simulink subsystem "LeastCov_v3_5_adaptiveAlgorithm"  (R2022a)
settings: Solver=VariableStepAuto  StartTime=0.0  StopTime=10.0  RelTol=1e-3
libraries: simulink x2
settings Model: Creator=targi  LastModifiedBy=targi

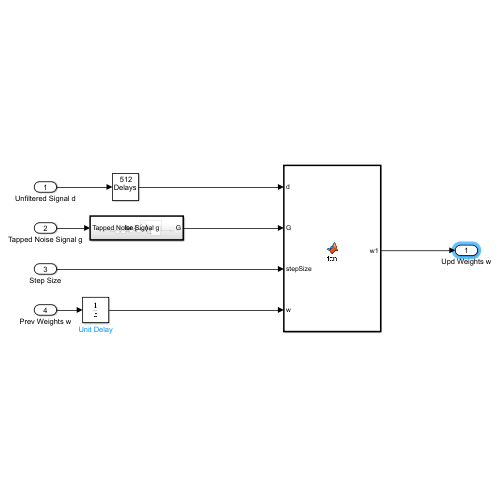
[thumbnail: Simulink's stored preview of the top-level diagram]
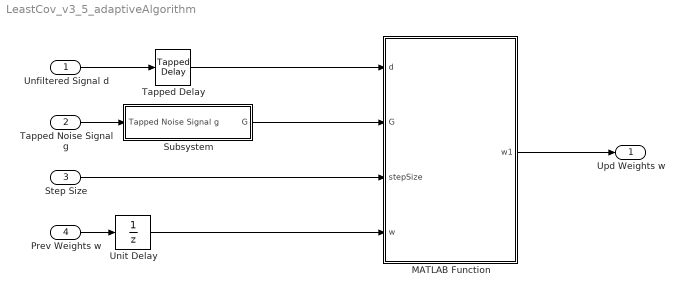
== system LeastCov_v3_5_adaptiveAlgorithm ==
  Unfiltered Signal d : Inport
  Tapped Noise Signal g : Inport  Port=2
  Step Size : Inport  Port=3
  Prev Weights w : Inport  Port=4
  MATLAB Function : MATLAB Function  TreatAsAtomicUnit=on
  Subsystem : Subsystem
  Tapped Delay : simulink/Discrete/Tapped Delay  vinit=0.0  samptime=-1  NumDelays=512  DelayOrder=Oldest  includeCurrent=off
  Unit Delay : UnitDelay  SampleTime=-1  HasFrameUpgradeWarning=on
  Upd Weights w : Outport
  wires:
  Tapped Noise Signal g/1 -> Subsystem/1(Tapped Noise Signal g)
  Prev Weights w/1 -> Unit Delay/1
  Unfiltered Signal d/1 -> Tapped Delay/1
  Unit Delay/1 -> MATLAB Function/4(w)
  Step Size/1 -> MATLAB Function/3(stepSize)
  Subsystem/1(G) -> MATLAB Function/2(G)
  Tapped Delay/1 -> MATLAB Function/1(d)
  MATLAB Function/1(w1) -> Upd Weights w/1

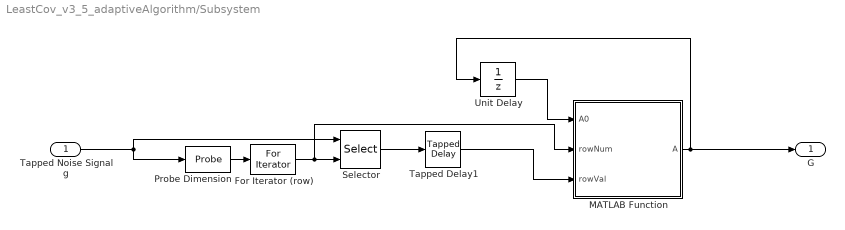
== system LeastCov_v3_5_adaptiveAlgorithm/Subsystem ==
  Tapped Noise Signal g : Inport
  For Iterator (row) : ForIterator  IterationSource=external
  MATLAB Function : MATLAB Function  TreatAsAtomicUnit=on
  Probe Dimension : Probe  ProbeSampleTime=off  ProbeComplexSignal=off
  Selector : Selector  IndexOptions=Starting index (port)  Indices=[1 3]  OutputSizes=1
  Tapped Delay1 : simulink/Discrete/Tapped Delay  vinit=0.0  samptime=-1  NumDelays=512  DelayOrder=Oldest  includeCurrent=off
  Unit Delay : UnitDelay  InitialCondition=zeros(256,512)  SampleTime=-1  HasFrameUpgradeWarning=on
  G : Outport
  wires:
  Unit Delay/1 -> MATLAB Function/1(A0)
  Tapped Delay1/1 -> MATLAB Function/3(rowVal)
  MATLAB Function/1(A) -> G/1, Unit Delay/1
  For Iterator (row)/1 -> Selector/2, MATLAB Function/2(rowNum)
  Probe Dimension/1 -> For Iterator (row)/1
  Tapped Noise Signal g/1 -> Selector/1, Probe Dimension/1
  Selector/1 -> Tapped Delay1/1

== matlab function LeastCov_v3_5_adaptiveAlgorithm/Subsystem/MATLAB Function ==
  data: A0 input; A output; rowNum input; rowVal input
function A = buildMatrix(A0, rowNum, rowVal)

A0(rowNum, :) = rowVal;
A = A0;

== matlab function LeastCov_v3_5_adaptiveAlgorithm/MATLAB Function ==
  data: d input; w1 output; G input; stepSize input; w input
function w1 = fcn(d, G, stepSize, w)

T = length(d);

A = d - 2*w'*G;
B = G*A';
C = sum(A,2) * sum(G,2);
D = (1/T)*B - ((1/T)^2)*C;

w1 = stepSize*D;
